simulink model "gm_parallel_lht"  (R2019b)
settings: Solver=FixedStepDiscrete  StartTime=0.0  StopTime=inf  RelTol=1e-3
undefined symbols (not defined in the file or in its folder): bt, height, width
libraries: hdlsllib x190, simulink x13, hdlmdlgenlib x7, dspsrcs4 x1
(part 1 of 18)
settings Model: SimulationMode=accelerator  Creator=rgb11127  LastModifiedBy=rgb11127
settings DataIOCC: SaveOutput=off  SaveTime=off
settings OptimizationCC: BlockReduction=off  ConditionallyExecuteInputs=off  DefaultParameterBehavior=Inlined
settings DebuggingCC: AlgebraicLoopMsg=error  InheritedTsInSrcMsg=none  SingleTaskRateTransMsg=error
settings HardwareCC: ProdBitPerPointer=32  ProdBitPerSizeT=32  ProdBitPerPtrDiffT=32  ProdLargestAtomicFloat=None  ProdIntDivRoundTo=Undefined  ProdEndianess=Unspecified  ProdWordSize=32  ProdHWDeviceType=ASIC/FPGA->ASIC/FPGA  TargetBitPerPointer=64  TargetBitPerSizeT=64  TargetBitPerPtrDiffT=64  TargetLongLongMode=on  TargetIntDivRoundTo=Zero  TargetEndianess=LittleEndian  TargetWordSize=64  TargetHWDeviceType=Custom Processor->MATLAB Host Computer  ProdEqTarget=off

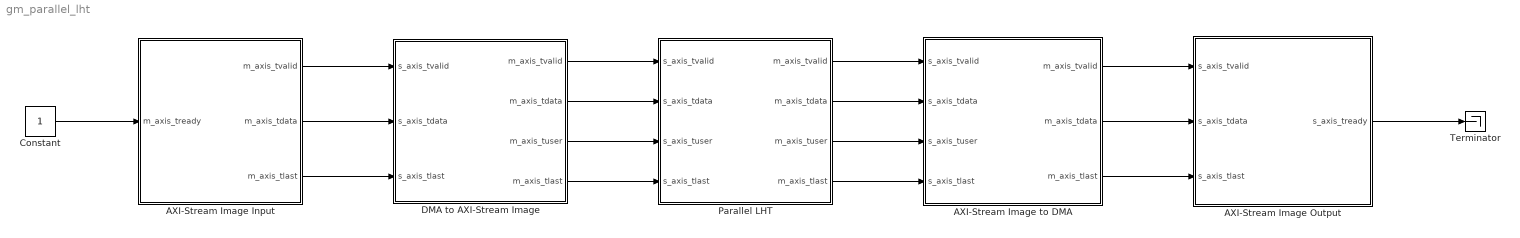
== system gm_parallel_lht ==
  AXI-Stream Image Input : Subsystem  mask{image=bt.inputImage, clk=1/150e6}
      mask prompts: image "Input Image:"; clk "Clock Rate:"
      mask init:
      | [height, width] = size(image);
      mask DialogControl DescGroupVar Prompt: AXI-Stream Image Input
      mask DialogControl DescTextVar Prompt: This block simulates an AXI-Stream image input for interfacing to a hardware accelerator or IP Core.
      mask DialogControl ParameterGroupVar Prompt: Main
  AXI-Stream Image Output : Subsystem  mask{height=bt.nRho, width=bt.nTheta, clk=1/150e6, d=0}
      mask prompts: height "Image Height:"; width "Image Width:"; clk "Clock Rate:"; d "Frame Capture Number"
      mask DialogControl DescGroupVar Prompt: AXI-Stream Image Output
      mask DialogControl DescTextVar Prompt: Image output using the AXI-Stream interface. Simulates an AXI DMA write channel.
      mask DialogControl ParameterGroupVar Prompt: Main
  AXI-Stream Image to DMA : Subsystem  mask{height=bt.nRho, width=bt.nTheta}
      mask prompts: height "Image Height"; width "Image Width"
      mask DialogControl DescGroupVar Prompt: AXI-Stream Image to DMA
      mask DialogControl DescTextVar Prompt: Converts from the AXI-Stream video standard to AXI-Stream DMA packet.
      mask DialogControl Container2 Prompt: Main
  Constant : Constant  OutDataTypeStr=boolean  SampleTime=-1
  DMA to AXI-Stream Image : Subsystem  mask{height=bt.height, width=bt.width, b=1}
      mask prompts: height "Image Height:"; width "Image Width:"; b "Bits"
      mask DialogControl DescGroupVar Prompt: DMA to AXI-Stream Image
      mask DialogControl DescTextVar Prompt: Converts an DMA AXI-Stream packet to the AXI-Stream video standard.
      mask DialogControl Container2 Prompt: Main
  Parallel LHT : Subsystem
  Terminator : Terminator
  wires:
  Parallel LHT/4(m_axis_tlast) -> AXI-Stream Image to DMA/4(s_axis_tlast)
  Parallel LHT/3(m_axis_tuser) -> AXI-Stream Image to DMA/3(s_axis_tuser)
  Parallel LHT/2(m_axis_tdata) -> AXI-Stream Image to DMA/2(s_axis_tdata)
  Parallel LHT/1(m_axis_tvalid) -> AXI-Stream Image to DMA/1(s_axis_tvalid)
  DMA to AXI-Stream Image/4(m_axis_tlast) -> Parallel LHT/4(s_axis_tlast)
  DMA to AXI-Stream Image/3(m_axis_tuser) -> Parallel LHT/3(s_axis_tuser)
  DMA to AXI-Stream Image/2(m_axis_tdata) -> Parallel LHT/2(s_axis_tdata)
  DMA to AXI-Stream Image/1(m_axis_tvalid) -> Parallel LHT/1(s_axis_tvalid)
  AXI-Stream Image Output/1(s_axis_tready) -> Terminator/1
  AXI-Stream Image to DMA/3(m_axis_tlast) -> AXI-Stream Image Output/3(s_axis_tlast)
  AXI-Stream Image to DMA/2(m_axis_tdata) -> AXI-Stream Image Output/2(s_axis_tdata)
  AXI-Stream Image to DMA/1(m_axis_tvalid) -> AXI-Stream Image Output/1(s_axis_tvalid)
  AXI-Stream Image Input/3(m_axis_tlast) -> DMA to AXI-Stream Image/3(s_axis_tlast)
  AXI-Stream Image Input/2(m_axis_tdata) -> DMA to AXI-Stream Image/2(s_axis_tdata)
  AXI-Stream Image Input/1(m_axis_tvalid) -> DMA to AXI-Stream Image/1(s_axis_tvalid)
  Constant/1 -> AXI-Stream Image Input/1(m_axis_tready)

== system gm_parallel_lht/AXI-Stream Image Input ==
  m_axis_tready : Inport
  Compare To Constant : simulink/Logic and Bit Operations/Compare To Constant  relop===  const=height*width-1  OutDataTypeStr=boolean
  Data Type Conversion : DataTypeConversion  OutDataTypeStr=uint32
  HDL Counter : hdlsllib/Sources/HDL Counter  CountType=Count limited  CountInit=0  CountStep=1  CountMax=width*height-1  CountFromType=Initial value  CountFrom=0  CountResetPort=off  CountLoadPort=off  CountEnbPort=on  CountDirPort=off  CountDataType=Unsigned  CountWordLen=ceil(log2(width*height))  CountFracLen=0  CountSampTime=1
      settings: SourceProductName=Simulink
  Master AXI-Stream FIFO : Subsystem  mask{depth=32}
      mask prompts: depth "FIFO Depth:"
      mask DialogControl DescGroupVar Prompt: Master AXI-Stream FIFO
      mask DialogControl DescTextVar Prompt: A custom AXI-Stream FIFO for interfacing to write channel AXI DMAs.
      mask DialogControl ParameterGroupVar Prompt: Main
  Synchronous Image Source : Subsystem
  m_axis_tvalid : Outport
  m_axis_tdata : Outport  Port=2
  m_axis_tlast : Outport  Port=3
  wires:
  HDL Counter/1 -> Compare To Constant/1
  Synchronous Image Source/1(Pixel) -> Data Type Conversion/1
  Master AXI-Stream FIFO/1(m_axis_tvalid) -> m_axis_tvalid/1
  Data Type Conversion/1 -> Master AXI-Stream FIFO/2(s_axis_tdata)
  Compare To Constant/1 -> Master AXI-Stream FIFO/3(s_axis_tlast)
  Master AXI-Stream FIFO/4(s_axis_tready) -> Synchronous Image Source/Enable, Master AXI-Stream FIFO/1(s_axis_tvalid), HDL Counter/1
  m_axis_tready/1 -> Master AXI-Stream FIFO/4(m_axis_tready)
  Master AXI-Stream FIFO/3(m_axis_tlast) -> m_axis_tlast/1
  Master AXI-Stream FIFO/2(m_axis_tdata) -> m_axis_tdata/1

== system gm_parallel_lht/AXI-Stream Image Output ==
  s_axis_tvalid : Inport
  s_axis_tdata : Inport  Port=2
  s_axis_tlast : Inport  Port=3
  AND1 : Logic  IconShape=distinctive  AllPortsSameDT=off  OutDataTypeStr=boolean
  Compare To Constant4 : simulink/Logic and Bit Operations/Compare To Constant  relop===  const=(height)*width-1  OutDataTypeStr=boolean
  Constant : Constant  OutDataTypeStr=boolean  SampleTime=-1
  Delay2 : Delay  DelayLength=d  ShowEnablePort=on
      settings: InputPortMap=u0,e6
  Pixel to Workspace : Subsystem
  Stop Simulation1 : Stop
  Terminator : Terminator
  Total Samples Counter : hdlsllib/Sources/HDL Counter  CountType=Count limited  CountInit=0  CountStep=1  CountMax=(height)*width-1  CountFromType=Initial value  CountFrom=0  CountResetPort=off  CountLoadPort=off  CountEnbPort=on  CountDirPort=off  CountDataType=Unsigned  CountWordLen=ceil(log2((height)*width+1))  CountFracLen=0  CountSampTime=1
      settings: SourceProductName=Simulink
  s_axis_tready : Outport  VectorParamsAs1DForOutWhenUnconnected=off
  wires:
  Constant/1 -> s_axis_tready/1, AND1/2
  s_axis_tlast/1 -> Terminator/1
  Delay2/1 -> Stop Simulation1/1
  Compare To Constant4/1 -> Delay2/1, Delay2/2
  Total Samples Counter/1 -> Compare To Constant4/1
  AND1/1 -> Pixel to Workspace/Enable, Total Samples Counter/1
  s_axis_tvalid/1 -> AND1/1
  s_axis_tdata/1 -> Pixel to Workspace/1(Pixel In)

== system gm_parallel_lht/AXI-Stream Image to DMA ==
  s_axis_tvalid : Inport
  s_axis_tdata : Inport  Port=2
  s_axis_tuser : Inport  Port=3
  s_axis_tlast : Inport  Port=4
  AND : Logic  IconShape=distinctive  AllPortsSameDT=off  OutDataTypeStr=boolean
  Compare To Constant : simulink/Logic and Bit Operations/Compare To Constant  relop===  const=height*width-1  OutDataTypeStr=boolean
  Data Type Conversion : DataTypeConversion  OutDataTypeStr=uint32
  Output Counter : hdlsllib/Sources/HDL Counter  CountType=Count limited  CountInit=0  CountStep=1  CountMax=height*width-1  CountFromType=Initial value  CountFrom=0  CountResetPort=off  CountLoadPort=off  CountEnbPort=on  CountDirPort=off  CountDataType=Unsigned  CountWordLen=ceil(log2(height*width))  CountFracLen=0  CountSampTime=1
      settings: SourceProductName=Simulink
  Terminator : Terminator
  Terminator1 : Terminator
  m_axis_tvalid : Outport
  m_axis_tdata : Outport  Port=2
  m_axis_tlast : Outport  Port=3
  wires:
  Data Type Conversion/1 -> m_axis_tdata/1
  s_axis_tdata/1 -> Data Type Conversion/1
  s_axis_tvalid/1 -> AND/2, m_axis_tvalid/1, Output Counter/1
  s_axis_tlast/1 -> Terminator/1
  s_axis_tuser/1 -> Terminator1/1
  Output Counter/1 -> Compare To Constant/1
  Compare To Constant/1 -> AND/1
  AND/1 -> m_axis_tlast/1

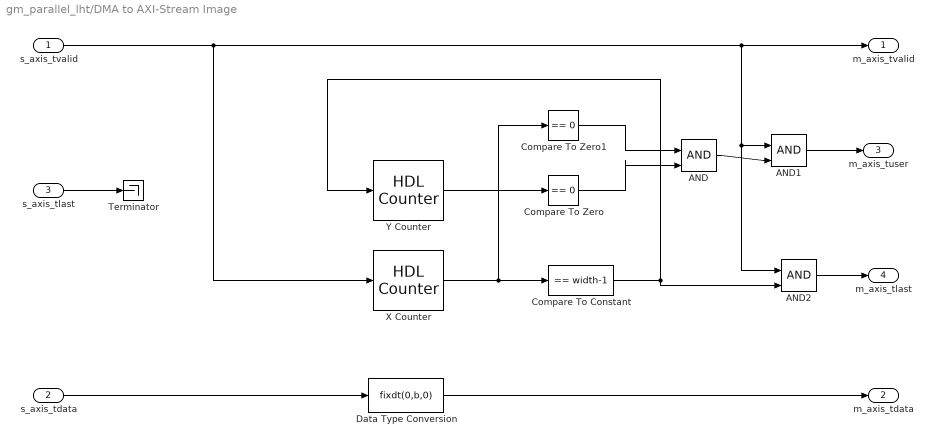
== system gm_parallel_lht/DMA to AXI-Stream Image ==
  s_axis_tvalid : Inport
  s_axis_tdata : Inport  Port=2
  s_axis_tlast : Inport  Port=3
  AND : Logic  IconShape=distinctive  AllPortsSameDT=off  OutDataTypeStr=boolean
  AND1 : Logic  IconShape=distinctive  AllPortsSameDT=off  OutDataTypeStr=boolean
  AND2 : Logic  IconShape=distinctive  AllPortsSameDT=off  OutDataTypeStr=boolean
  Compare To Constant : simulink/Logic and Bit Operations/Compare To Constant  relop===  const=width-1  OutDataTypeStr=boolean
  Compare To Zero : simulink/Logic and Bit Operations/Compare To Zero  relop===  OutDataTypeStr=boolean
  Compare To Zero1 : simulink/Logic and Bit Operations/Compare To Zero  relop===  OutDataTypeStr=boolean
  Data Type Conversion : DataTypeConversion  OutDataTypeStr=fixdt(0,b,0)  ConvertRealWorld=Stored Integer (SI)
  Terminator : Terminator
  X Counter : hdlsllib/Sources/HDL Counter  CountType=Count limited  CountInit=0  CountStep=1  CountMax=width-1  CountFromType=Initial value  CountFrom=0  CountResetPort=off  CountLoadPort=off  CountEnbPort=on  CountDirPort=off  CountDataType=Unsigned  CountWordLen=ceil(log2(width))  CountFracLen=0  CountSampTime=1
      settings: SourceProductName=Simulink
  Y Counter : hdlsllib/Sources/HDL Counter  CountType=Count limited  CountInit=0  CountStep=1  CountMax=height-1  CountFromType=Initial value  CountFrom=0  CountResetPort=off  CountLoadPort=off  CountEnbPort=on  CountDirPort=off  CountDataType=Unsigned  CountWordLen=ceil(log2(height))  CountFracLen=0  CountSampTime=1
      settings: SourceProductName=Simulink
  m_axis_tvalid : Outport
  m_axis_tdata : Outport  Port=2
  m_axis_tuser : Outport  Port=3
  m_axis_tlast : Outport  Port=4
  wires:
  s_axis_tlast/1 -> Terminator/1
  Data Type Conversion/1 -> m_axis_tdata/1
  s_axis_tvalid/1 -> X Counter/1, AND2/1, AND1/1, m_axis_tvalid/1
  X Counter/1 -> Compare To Zero1/1, Compare To Constant/1
  Y Counter/1 -> Compare To Zero/1
  Compare To Zero1/1 -> AND/1
  Compare To Zero/1 -> AND/2
  s_axis_tdata/1 -> Data Type Conversion/1
  AND/1 -> AND1/2
  AND1/1 -> m_axis_tuser/1
  Compare To Constant/1 -> AND2/2, Y Counter/1
  AND2/1 -> m_axis_tlast/1

== system gm_parallel_lht/Parallel LHT ==
  s_axis_tvalid : Inport  OutDataTypeStr=boolean  PortDimensions=1  SampleTime=6.66666666666667e-09
  s_axis_tdata : Inport  Port=2  OutDataTypeStr=fixdt(0, 1, 0)  PortDimensions=1  SampleTime=6.66666666666667e-09
  s_axis_tuser : Inport  Port=3  OutDataTypeStr=boolean  PortDimensions=1  SampleTime=6.66666666666667e-09
  s_axis_tlast : Inport  Port=4  OutDataTypeStr=boolean  PortDimensions=1  SampleTime=6.66666666666667e-09
  Parallel LHT Accumulator : Subsystem  mask{height=double(768), width=double(1024), theta=reshape(double([0 1 2 3 4 5 6 7 8 9 10 11 12 13 14 15 16 17 18 19 20 21 22 23 24 25 26 27 28 29 30 31 32 33 34 35 36 37 38 39 40 41 42 43 44 45 46 47 48 49 50 51 52 53 54 55 56 57 58 59 60 61 62 63 64 65 66 67 68 69 70 71 72 73 74 75 76 77 78 79 80 81 82 83 84 85 86 87 88 89 90 91 92 93 94 95 96 97 98 99 100 101 102 103 104 105 106 107 108 109 110 111 112 113 114 115 116 117 118 119 120 121 122 123 124 125 126 127 128 129 130 131 132 133 134 135 136 137 138 139 140 141 142 143 144 145 146 147 148 149 150 151 152 153 154 155 156 157 158 159 160 161 162 163 164 165 166 167 168 169 170 171 172 173 174 175 176 177 178 179]).', [1  180])}
      mask prompts: height "Image Height:"; width "Image Width:"; theta "Orientations:"
      mask init:
      | maxRho = ceil(sqrt((height/2)^2+(width/2)^2));
      | nRho = maxRho*2;
      | [~, nTheta] = size(theta);
  Parallel LHT Kernel : Subsystem  mask{height=double(768), width=double(1024), theta=reshape(double([0 1 2 3 4 5 6 7 8 9 10 11 12 13 14 15 16 17 18 19 20 21 22 23 24 25 26 27 28 29 30 31 32 33 34 35 36 37 38 39 40 41 42 43 44 45 46 47 48 49 50 51 52 53 54 55 56 57 58 59 60 61 62 63 64 65 66 67 68 69 70 71 72 73 74 75 76 77 78 79 80 81 82 83 84 85 86 87 88 89 90 91 92 93 94 95 96 97 98 99 100 101 102 103 104 105 106 107 108 109 110 111 112 113 114 115 116 117 118 119 120 121 122 123 124 125 126 127 128 129 130 131 132 133 134 135 136 137 138 139 140 141 142 143 144 145 146 147 148 149 150 151 152 153 154 155 156 157 158 159 160 161 162 163 164 165 166 167 168 169 170 171 172 173 174 175 176 177 178 179]).', [1  180]), kFlag=Symmetric Look Ahead}
      mask prompts: height "Image Height:"; width "Image Width:"; theta "Orientations:"; kFlag "Kernel Architecture:"
      mask init:
      | maxRho = ceil(sqrt((height/2)^2+(width/2)^2));
      | [~, nTheta] = size(theta);
      | nRho = maxRho*2;
      | 
      | blk = [gcb '/Hough Kernel'];
      | 
      | oldVariant = get_param(blk,'OverrideUsingVariant');
      | 
      | switch get_param(gcb, 'kFlag')
      |     case 'Parallel'
      |         newVariant = 'Parallel';
      |     case 'Symmetric'
      |         newVariant = 'Symmetric';
      |     case 'Symmetric Look Ahead'
      |         newVariant = 'SymmetricLookAhead';
      |     otherwise
      |         newVariant = 'Simple';
      | end
      | 
      | if ~strcmp(oldVariant, newVariant)
      |     set_param(blk, 'OverrideUsingVariant', newVariant);
      | end
      mask TypeOptions kFlag: Parallel | Symmetric | Symmetric Look Ahead
  delayMatch : Delay  DelayLength=double(2)  InitialCondition=0  SampleTime=6.66666666666667e-09
  delayMatch1 : Delay  DelayLength=double(2)  InitialCondition=0  SampleTime=6.66666666666667e-09
  delayMatch2 : Delay  DelayLength=double(2)  InitialCondition=0  SampleTime=6.66666666666667e-09
  m_axis_tvalid : Outport
  m_axis_tdata : Outport  Port=2
  m_axis_tuser : Outport  Port=3
  m_axis_tlast : Outport  Port=4
  wires:
  s_axis_tvalid/1 -> Parallel LHT Kernel/1(s_axis_tvalid)
  s_axis_tdata/1 -> Parallel LHT Kernel/2(s_axis_tdata)
  s_axis_tuser/1 -> Parallel LHT Kernel/3(s_axis_tuser)
  s_axis_tlast/1 -> Parallel LHT Kernel/4(s_axis_tlast)
  delayMatch/1 -> m_axis_tvalid/1
  Parallel LHT Accumulator/2(m_axis_tdata) -> m_axis_tdata/1
  delayMatch1/1 -> m_axis_tuser/1
  delayMatch2/1 -> m_axis_tlast/1
  Parallel LHT Kernel/1(m_axis_tvalid) -> Parallel LHT Accumulator/1(s_axis_tvalid)
  Parallel LHT Kernel/2(m_axis_tdata) -> Parallel LHT Accumulator/2(s_axis_tdata)
  Parallel LHT Kernel/3(m_axis_tuser) -> Parallel LHT Accumulator/3(s_axis_tuser)
  Parallel LHT Kernel/4(m_axis_tlast) -> Parallel LHT Accumulator/4(s_axis_tlast)
  Parallel LHT Kernel/5(hough_param) -> Parallel LHT Accumulator/5(hough_param)
  Parallel LHT Accumulator/1(m_axis_tvalid) -> delayMatch/1
  Parallel LHT Accumulator/3(m_axis_tuser) -> delayMatch1/1
  Parallel LHT Accumulator/4(m_axis_tlast) -> delayMatch2/1

== system gm_parallel_lht/AXI-Stream Image Input/Master AXI-Stream FIFO ==
  s_axis_tvalid : Inport
  s_axis_tdata : Inport  Port=2
  s_axis_tlast : Inport  Port=3
  m_axis_tready : Inport  Port=4
  AND : Logic  IconShape=distinctive  AllPortsSameDT=off  OutDataTypeStr=boolean
  "Compare To Constant " : simulink/Logic and Bit Operations/Compare To Constant  relop=>=  const=floor(depth/2)  OutDataTypeStr=boolean
  Delay : Delay  DelayLength=1
  HDL FIFO TDATA : hdlsllib/HDL RAMs/HDL FIFO  fifo_size=depth  mode=Classic  ratio=1  push_msg=Error  pop_msg=Error  show_empty=on  show_full=off  show_num=on  LabelModeActiveChoice_Mode=Classic
      settings: SourceProductName=Simulink  SourceProductBaseCode=SL
  HDL FIFO TLAST : hdlsllib/HDL RAMs/HDL FIFO  fifo_size=depth  mode=Classic  ratio=1  push_msg=Error  pop_msg=Error  show_empty=off  show_full=off  show_num=off  LabelModeActiveChoice_Mode=Classic
      settings: SourceProductName=Simulink  SourceProductBaseCode=SL
  NOT : Logic  Operator=NOT  IconShape=distinctive  AllPortsSameDT=off  OutDataTypeStr=boolean
  NOT1 : Logic  Operator=NOT  IconShape=distinctive  AllPortsSameDT=off  OutDataTypeStr=boolean
  m_axis_tvalid : Outport  VectorParamsAs1DForOutWhenUnconnected=off
  m_axis_tdata : Outport  Port=2  VectorParamsAs1DForOutWhenUnconnected=off
  m_axis_tlast : Outport  Port=3  VectorParamsAs1DForOutWhenUnconnected=off
  s_axis_tready : Outport  Port=4
  wires:
  HDL FIFO TDATA/1 -> m_axis_tdata/1
  HDL FIFO TLAST/1 -> m_axis_tlast/1
  HDL FIFO TDATA/2 -> NOT/1
  AND/1 -> HDL FIFO TLAST/3, HDL FIFO TDATA/3
  NOT/1 -> Delay/1, AND/2
  m_axis_tready/1 -> AND/1
  HDL FIFO TDATA/3 -> "Compare To Constant "/1
  NOT1/1 -> s_axis_tready/1
  "Compare To Constant "/1 -> NOT1/1
  s_axis_tlast/1 -> HDL FIFO TLAST/1
  s_axis_tdata/1 -> HDL FIFO TDATA/1
  s_axis_tvalid/1 -> HDL FIFO TLAST/2, HDL FIFO TDATA/2
  Delay/1 -> m_axis_tvalid/1

== system gm_parallel_lht/AXI-Stream Image Input/Synchronous Image Source ==
  Enable : EnablePort
  Signal From Workspace : dspsrcs4/Signal From Workspace  X=reshape(image', [height*width, 1])  Ts=clk  nsamps=1  OutputAfterFinalValue=Cyclic repetition  ignoreOrWarnInputAndFrameLengths=off  OutputFrames=off
  Pixel : Outport
  wires:
  Signal From Workspace/1 -> Pixel/1

== system gm_parallel_lht/AXI-Stream Image Output/Pixel to Workspace ==
  Pixel In : Inport
  Enable : EnablePort
  To Workspace : ToWorkspace  VariableName=simout  SampleTime=-1
      settings: MaxDataPoints=height*width  Save2DSignal=2-D array (concatenate along first dimension)
  wires:
  Pixel In/1 -> To Workspace/1

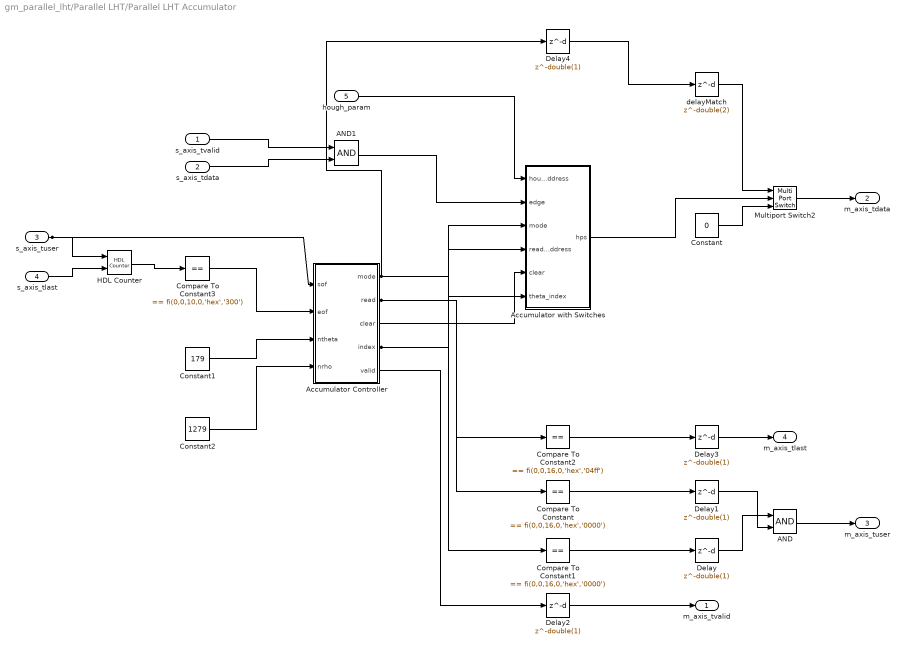
== system gm_parallel_lht/Parallel LHT/Parallel LHT Accumulator ==
  s_axis_tvalid : Inport  OutDataTypeStr=boolean  PortDimensions=1  SampleTime=6.66666666666667e-09
  s_axis_tdata : Inport  Port=2  OutDataTypeStr=fixdt(0, 1, 0)  PortDimensions=1  SampleTime=6.66666666666667e-09
  s_axis_tuser : Inport  Port=3  OutDataTypeStr=boolean  PortDimensions=1  SampleTime=6.66666666666667e-09
  s_axis_tlast : Inport  Port=4  OutDataTypeStr=boolean  PortDimensions=1  SampleTime=6.66666666666667e-09
  hough_param : Inport  Port=5  OutDataTypeStr=fixdt(0, 11, 0)  PortDimensions=[1 180]  SampleTime=6.66666666666667e-09
  AND : Logic  AllPortsSameDT=off  OutDataTypeStr=boolean  SampleTime=6.66666666666667e-09
  AND1 : Logic  AllPortsSameDT=off  OutDataTypeStr=boolean  SampleTime=6.66666666666667e-09
  Accumulator Controller : Subsystem
  Accumulator with Switches : Subsystem
  Compare To Constant : simulink/Logic and Bit Operations/Compare To Constant  relop===  const=fi(0,0,16,0,'hex','0000')  OutDataTypeStr=boolean
  Compare To Constant1 : simulink/Logic and Bit Operations/Compare To Constant  relop===  const=fi(0,0,16,0,'hex','0000')  OutDataTypeStr=boolean
  Compare To Constant2 : simulink/Logic and Bit Operations/Compare To Constant  relop===  const=fi(0,0,16,0,'hex','04ff')  OutDataTypeStr=boolean
  Compare To Constant3 : simulink/Logic and Bit Operations/Compare To Constant  relop===  const=fi(0,0,10,0,'hex','300')  OutDataTypeStr=boolean
  Constant : Constant  Value=0  OutDataTypeStr=fixdt(0, 11, 0)  SampleTime=-1
  Constant1 : Constant  Value=179  OutDataTypeStr=uint16  SampleTime=-1
  Constant2 : Constant  Value=1279  OutDataTypeStr=uint16  SampleTime=-1
  Delay{,1..4} (5 alike) : Delay  DelayLength=double(1)  InitialCondition=0  SampleTime=6.66666666666667e-09
  HDL Counter : hdlsllib/Sources/HDL Counter  CountType=Count limited  CountInit=double(0)  CountStep=double(1)  CountMax=double(768)  CountFromType=Initial value  CountFrom=double(0)  CountResetPort=on  CountLoadPort=off  CountEnbPort=on  CountDirPort=off  CountDataType=Unsigned  CountWordLen=10  CountFracLen=0  CountSampTime=6.66666666666667e-09
      settings: SourceProductName=Simulink
  Multiport Switch2 : MultiPortSwitch  DataPortOrder=Zero-based contiguous  Inputs=2  DiagnosticForDefault=None  zeroidx=on  OutDataTypeStr=fixdt(0, 11, 0)  SampleTime=6.66666666666667e-09
  delayMatch : Delay  DelayLength=double(2)  InitialCondition=0  SampleTime=6.66666666666667e-09
  m_axis_tvalid : Outport
  m_axis_tdata : Outport  Port=2
  m_axis_tuser : Outport  Port=3
  m_axis_tlast : Outport  Port=4
  wires:
  AND/1 -> m_axis_tuser/1
  AND1/1 -> Accumulator with Switches/2(edge)
  Accumulator Controller/1(mode) -> Delay4/1, Accumulator with Switches/3(mode)
  Accumulator Controller/2(read) -> Compare To Constant2/1, Compare To Constant/1, Accumulator with Switches/4(read_address)
  Accumulator Controller/3(clear) -> Accumulator with Switches/5(clear)
  Accumulator Controller/4(index) -> Compare To Constant1/1, Accumulator with Switches/6(theta_index)
  Accumulator Controller/5(valid) -> Delay2/1
  Accumulator with Switches/1(hps) -> Multiport Switch2/2
  Compare To Constant/1 -> Delay1/1
  Compare To Constant1/1 -> Delay/1
  Compare To Constant2/1 -> Delay3/1
  Compare To Constant3/1 -> Accumulator Controller/2(eof)
  Constant/1 -> Multiport Switch2/3
  Constant1/1 -> Accumulator Controller/3(ntheta)
  Constant2/1 -> Accumulator Controller/4(nrho)
  Delay/1 -> AND/1
  Delay1/1 -> AND/2
  Delay2/1 -> m_axis_tvalid/1
  Delay3/1 -> m_axis_tlast/1
  delayMatch/1 -> Multiport Switch2/1
  HDL Counter/1 -> Compare To Constant3/1
  Multiport Switch2/1 -> m_axis_tdata/1
  s_axis_tvalid/1 -> AND1/1
  s_axis_tdata/1 -> AND1/2
  s_axis_tuser/1 -> HDL Counter/1, Accumulator Controller/1(sof)
  s_axis_tlast/1 -> HDL Counter/2
  hough_param/1 -> Accumulator with Switches/1(hough_address)
  Delay4/1 -> delayMatch/1

== system gm_parallel_lht/Parallel LHT/Parallel LHT Kernel ==
  s_axis_tvalid : Inport  OutDataTypeStr=boolean  PortDimensions=1  SampleTime=6.66666666666667e-09
  s_axis_tdata : Inport  Port=2  OutDataTypeStr=fixdt(0, 1, 0)  PortDimensions=1  SampleTime=6.66666666666667e-09
  s_axis_tuser : Inport  Port=3  OutDataTypeStr=boolean  PortDimensions=1  SampleTime=6.66666666666667e-09
  s_axis_tlast : Inport  Port=4  OutDataTypeStr=boolean  PortDimensions=1  SampleTime=6.66666666666667e-09
  AND : Logic  IconShape=distinctive  AllPortsSameDT=off  OutDataTypeStr=boolean
  Add1 : Sum  OutDataTypeStr=fixdt(0, ceil(log2(2*maxRho+1)), 0);  RndMeth=Round
  Constant1 : Constant  Value=maxRho  OutDataTypeStr=fixdt(0, ceil(log2(maxRho + 1)), 0);  SampleTime=-1
  Hough Kernel : Subsystem
  X Counter : hdlsllib/Sources/HDL Counter  CountType=Count limited  CountInit=-width/2  CountStep=1  CountMax=width/2-1  CountFromType=Initial value  CountFrom=-width/2  CountResetPort=off  CountLoadPort=off  CountEnbPort=on  CountDirPort=off  CountDataType=Signed  CountWordLen=ceil(log2(width))  CountFracLen=0  CountSampTime=1
      settings: SourceProductName=Simulink
  Y Counter : hdlsllib/Sources/HDL Counter  CountType=Count limited  CountInit=-height/2  CountStep=1  CountMax=height/2-1  CountFromType=Initial value  CountFrom=-height/2  CountResetPort=off  CountLoadPort=off  CountEnbPort=on  CountDirPort=off  CountDataType=Signed  CountWordLen=ceil(log2(height))  CountFracLen=0  CountSampTime=1
      settings: SourceProductName=Simulink
  m_axis_tvalid : Outport
  m_axis_tdata : Outport  Port=2
  m_axis_tuser : Outport  Port=3
  m_axis_tlast : Outport  Port=4
  hough_param : Outport  Port=5
  wires:
  AND/1 -> Y Counter/1
  Add1/1 -> hough_param/1
  Constant1/1 -> Add1/1
  Hough Kernel/1(Rho) -> Add1/2
  X Counter/1 -> Hough Kernel/1(X)
  Y Counter/1 -> Hough Kernel/2(Y)
  s_axis_tvalid/1 -> AND/1, X Counter/1, m_axis_tvalid/1
  s_axis_tdata/1 -> m_axis_tdata/1
  s_axis_tuser/1 -> m_axis_tuser/1
  s_axis_tlast/1 -> AND/2, m_axis_tlast/1

== system gm_parallel_lht/Parallel LHT/Parallel LHT Accumulator/Accumulator Controller ==
  sof : Inport  OutDataTypeStr=boolean  PortDimensions=1  SampleTime=6.66666666666667e-09
  eof : Inport  Port=2  OutDataTypeStr=boolean  PortDimensions=1  SampleTime=6.66666666666667e-09
  ntheta : Inport  Port=3  OutDataTypeStr=uint16  PortDimensions=1  SampleTime=6.66666666666667e-09
  nrho : Inport  Port=4  OutDataTypeStr=uint16  PortDimensions=1  SampleTime=6.66666666666667e-09
  Accumulator Controller : MATLAB Function  TreatAsAtomicUnit=on
  mode : Outport
  read : Outport  Port=2
  clear : Outport  Port=3
  index : Outport  Port=4
  valid : Outport  Port=5
  wires:
  Accumulator Controller/1(mode) -> mode/1
  Accumulator Controller/2(read) -> read/1
  Accumulator Controller/3(clear) -> clear/1
  Accumulator Controller/4(index) -> index/1
  Accumulator Controller/5(valid) -> valid/1
  sof/1 -> Accumulator Controller/1(sof)
  eof/1 -> Accumulator Controller/2(eof)
  ntheta/1 -> Accumulator Controller/3(ntheta)
  nrho/1 -> Accumulator Controller/4(nrho)
